simulink model "controlador_trolley"  (R2023b)
settings: Solver=FixedStepAuto  StartTime=0.0  StopTime=10.0  RelTol=1e-3
undefined symbols (not defined in the file): DiscIntNeverNeededParam, Kd_t, Ki_t, Kp_t, T_s2
settings Model: Creator=renzo  LastModifiedBy=Ferran

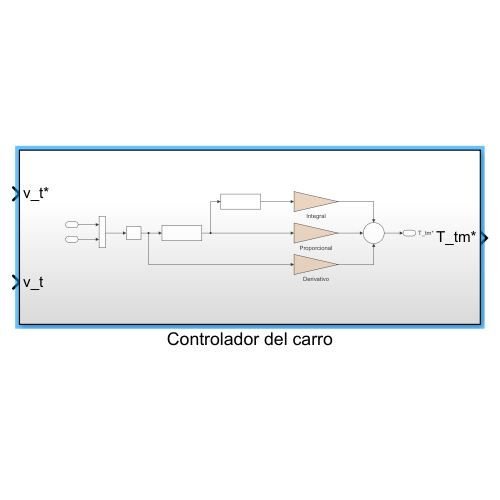
[thumbnail: Simulink's stored preview of the top-level diagram]
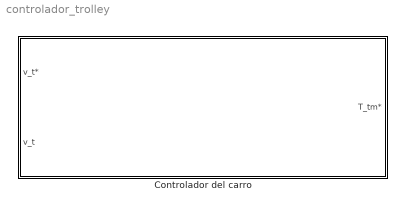
== system controlador_trolley ==
  Controlador del carro : Subsystem

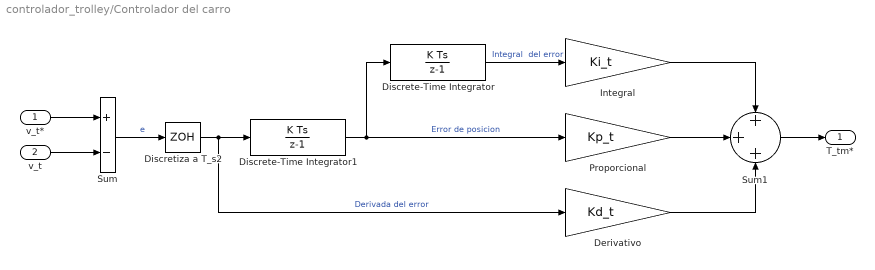
== system controlador_trolley/Controlador del carro ==
  v_t* : Inport
  v_t : Inport  Port=2
  Derivativo : Gain  Gain=Kd_t
  Discrete-Time Integrator : DiscreteIntegrator  SampleTime=T_s2  ICPrevOutput=DiscIntNeverNeededParam  ICPrevScaledInput=DiscIntNeverNeededParam
  Discrete-Time Integrator1 : DiscreteIntegrator  SampleTime=T_s2  ICPrevOutput=DiscIntNeverNeededParam  ICPrevScaledInput=DiscIntNeverNeededParam
  Discretiza a T_s2 : ZeroOrderHold  SampleTime=T_s2
  Integral : Gain  Gain=Ki_t
  Proporcional : Gain  Gain=Kp_t
  Sum : Sum  Inputs=+-
  Sum1 : Sum  Inputs=+++
  T_tm* : Outport
  wires:
  Discrete-Time Integrator1/1 -> Proporcional/1, Discrete-Time Integrator/1  "Error de posicion"
  v_t/1 -> Sum/2
  Discretiza a T_s2/1 -> Discrete-Time Integrator1/1, Derivativo/1  "Derivada del error"
  Sum/1 -> Discretiza a T_s2/1  "e"
  Derivativo/1 -> Sum1/3
  Integral/1 -> Sum1/1
  Sum1/1 -> T_tm*/1
  Discrete-Time Integrator/1 -> Integral/1  "Integral  del error"
  v_t*/1 -> Sum/1
  Proporcional/1 -> Sum1/2
